simulink model "phase_counter_tb2"  (R2019b)
settings: Solver=FixedStepDiscrete  StartTime=0.0  StopTime=500  RelTol=1e-3
libraries: dspsrcs4 x4, lib_dsphdlutils_v1 x2, lib_dsphdldsp_v1 x2, simulink x1
settings Model: DataTypeOverride=Off  Creator=mbabst  LastModifiedBy=mbabst
settings DataIOCC: SaveOutput=off  SaveTime=off
settings OptimizationCC: BlockReduction=off  ConditionallyExecuteInputs=off  DefaultParameterBehavior=Inlined
settings DebuggingCC: AlgebraicLoopMsg=error  SingleTaskRateTransMsg=error  ArithmeticOperatorsInVariantConditions=warning
settings HardwareCC: ProdBitPerPointer=32  ProdBitPerSizeT=32  ProdBitPerPtrDiffT=32  ProdLargestAtomicFloat=None  ProdIntDivRoundTo=Undefined  ProdEndianess=Unspecified  ProdWordSize=32  ProdHWDeviceType=ASIC/FPGA->ASIC/FPGA  ProdEqTarget=off
settings SFSimCC: SimUseLocalCustomCode=off  CustomCodeUndefinedFunction=UseInterfaceOnly
settings RTWCC: RTWUseLocalCustomCode=off
settings CodeAppCC: StateflowObjectComments=on

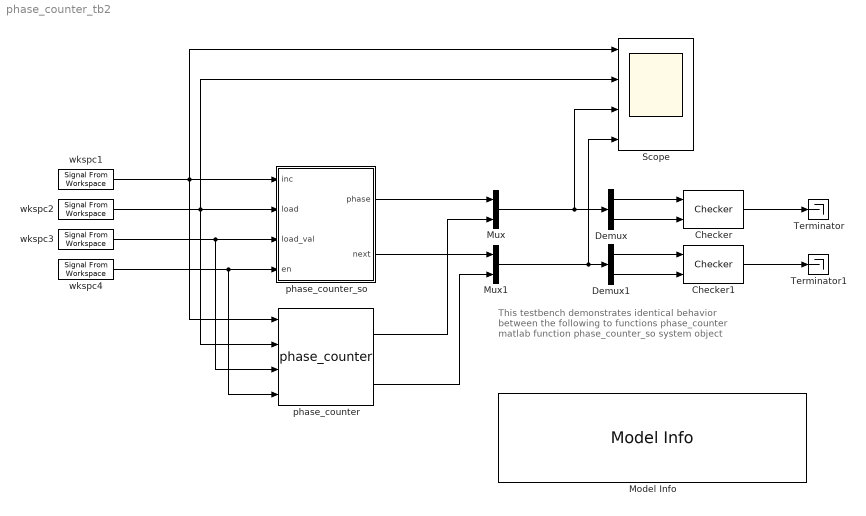
== system phase_counter_tb2 ==
  note: This testbench demonstrates identical behavior between the following to functions
      | phase_counter matlab function
      | phase_counter_so system object
  Checker : lib_dsphdlutils_v1/Checker  StopSim=on
      settings: SourceProductName=DSPHDL Library
  Checker1 : lib_dsphdlutils_v1/Checker  StopSim=on
      settings: SourceProductName=DSPHDL Library
  Demux : Demux  Outputs=2
  Demux1 : Demux  Outputs=2
  Model Info : simulink/Model-Wide Utilities/Model Info  Frame=on  DisplayStringWithTags=|  HorizontalTextAlignment=Left  LeftAlignmentValue=0.02
      | Copyright (c) 2005-2021 DSPlogic, Inc.
      | Distributed under the terms of the Simplified BSD License.
      | The full license is in the file LICENSE, distributed with this software.
      | 
      | Model: %<ModelName> (v%<ModelVersion>)
      | Author: Michael Babst <mike.babst@dsplogic.com>
      | Created: by %<Creator> on %<Created>
      | Modified: by %<ModifiedBy> on %<LastModificationDate>
  Mux : Mux  Inputs=2
  Mux1 : Mux  Inputs=2
  Scope : Scope  NumInputPorts=4
  Terminator : Terminator
  Terminator1 : Terminator
  phase_counter : lib_dsphdldsp_v1/phase_counter  SystemSampleTime=-1  Latency=0  AutoFrameSizeCalculation=off
  phase_counter_so : Subsystem
  wkspc1 : dspsrcs4/Signal From Workspace  X=inc  Ts=1  nsamps=1  OutputAfterFinalValue=Setting to zero  ignoreOrWarnInputAndFrameLengths=off  OutputFrames=off
  wkspc2 : dspsrcs4/Signal From Workspace  X=load  Ts=1  nsamps=1  OutputAfterFinalValue=Setting to zero  ignoreOrWarnInputAndFrameLengths=off  OutputFrames=off
  wkspc3 : dspsrcs4/Signal From Workspace  X=load_val  Ts=1  nsamps=1  OutputAfterFinalValue=Setting to zero  ignoreOrWarnInputAndFrameLengths=off  OutputFrames=off
  wkspc4 : dspsrcs4/Signal From Workspace  X=en  Ts=1  nsamps=1  OutputAfterFinalValue=Setting to zero  ignoreOrWarnInputAndFrameLengths=off  OutputFrames=off
  wires:
  wkspc1/1 -> phase_counter/1, phase_counter_so/1(inc), Scope/1
  wkspc2/1 -> phase_counter/2, phase_counter_so/2(load), Scope/2
  wkspc3/1 -> phase_counter/3, phase_counter_so/3(load_val)
  phase_counter_so/1(phase) -> Mux/1
  phase_counter/1 -> Mux/2
  Mux/1 -> Demux/1, Scope/3
  phase_counter_so/2(next) -> Mux1/1
  phase_counter/2 -> Mux1/2
  Mux1/1 -> Demux1/1, Scope/4
  Demux/1 -> Checker/1
  Demux/2 -> Checker/2
  Demux1/2 -> Checker1/2
  Demux1/1 -> Checker1/1
  Checker/1 -> Terminator/1
  Checker1/1 -> Terminator1/1
  wkspc4/1 -> phase_counter/4, phase_counter_so/4(en)

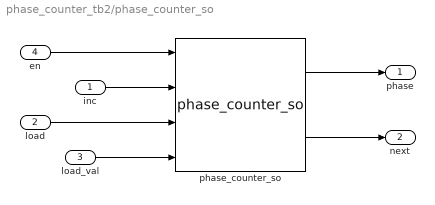
== system phase_counter_tb2/phase_counter_so ==
  inc : Inport
  load : Inport  Port=2
  load_val : Inport  Port=3
  en : Inport  Port=4
  phase_counter_so : lib_dsphdldsp_v1/phase_counter_so  WordLength=WordLength  SimulateUsing=Code generation
  phase : Outport
  next : Outport  Port=2
  wires:
  inc/1 -> phase_counter_so/2
  phase_counter_so/2 -> next/1
  phase_counter_so/1 -> phase/1
  load/1 -> phase_counter_so/3
  load_val/1 -> phase_counter_so/4
  en/1 -> phase_counter_so/1
